simulink model "tcm"  (Simulink 8.7)
settings: Solver=ode3  StartTime=0.0  StopTime=100.0  RelTol=1e-3
undefined symbols (not defined in the file or in its folder): ap, bias, sgn
libraries: simulink x3
settings Model: Creator=mddavies  LastModifiedBy=bourbouh
settings DataIOCC: SignalLoggingSaveFormat=ModelDataLogs
settings DebuggingCC: SolverPrmCheckMsg=warning  FcnCallInpInsideContextMsg=UseLocalSettings  StateNameClashWarn=warning
settings GRTTargetCC: CombineOutputUpdateFcns=off  GRTInterface=on

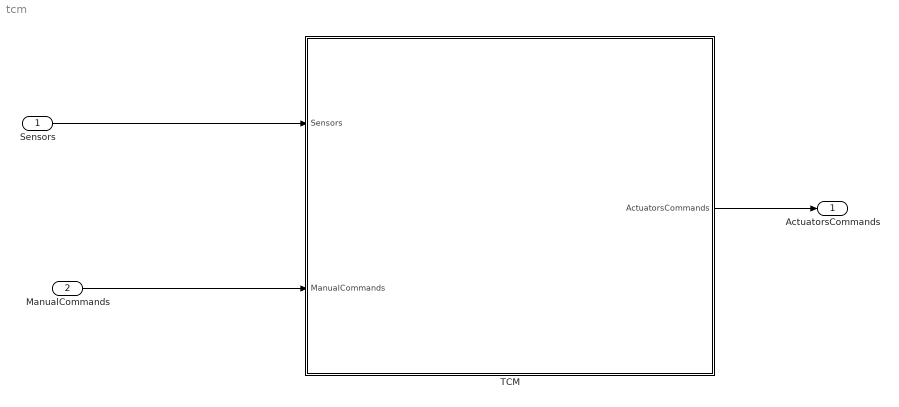
== system tcm ==
  Sensors : Inport  RequirementInfo={} %GIDa_0ce9b168_5661_42b0_b4cb_7d3faaf2df72  PortDimensions=17
  "ManualCommands " : Inport  RequirementInfo={} %GIDa_0ce9b168_5661_42b0_b4cb_7d3faaf2df72  Port=2  PortDimensions=9
  TCM : Subsystem
  ActuatorsCommands : Outport  RequirementInfo={} %GIDa_ba9bc9f0_2997_4cec_8a5a_2cb65716cddf
  wires:
  Sensors/1 -> TCM/1(Sensors)
  "ManualCommands "/1 -> TCM/2("ManualCommands ")
  TCM/1(ActuatorsCommands) -> ActuatorsCommands/1

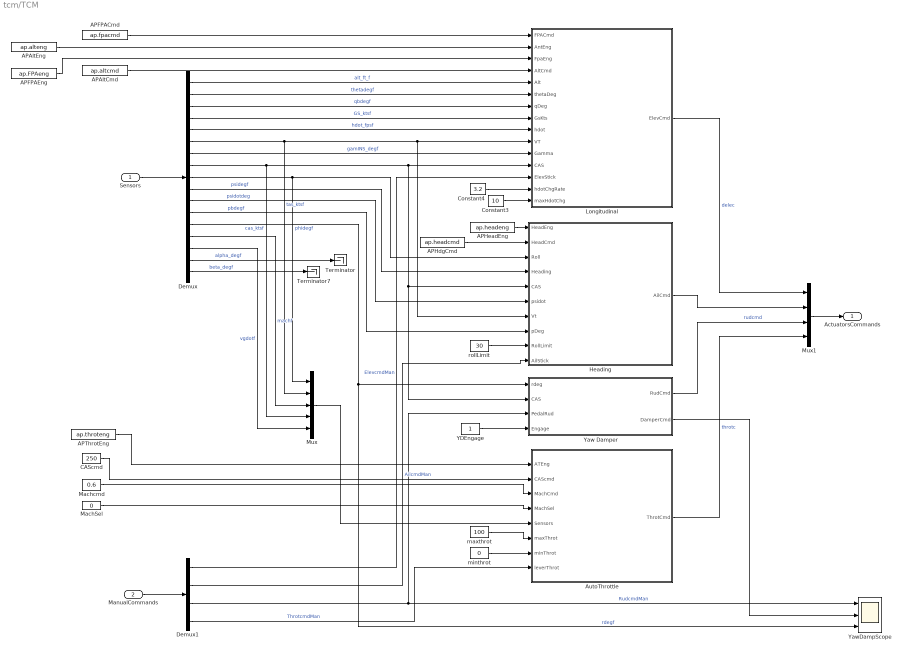
== system tcm/TCM ==
  Sensors : Inport  RequirementInfo={} %GIDa_0ce9b168_5661_42b0_b4cb_7d3faaf2df72  PortDimensions=17
  "ManualCommands " : Inport  RequirementInfo={} %GIDa_0ce9b168_5661_42b0_b4cb_7d3faaf2df72  Port=2  PortDimensions=9
  APAltCmd : Constant  RequirementInfo={} %GIDa_8396ea73_c2c1_410d_8e72_0a2c2e115229  Value=ap.altcmd
  APAltEng : Constant  RequirementInfo={} %GIDa_7acdc276_5904_4f5d_a4d8_b7eafc22dcba  Value=ap.alteng  OutDataTypeStr=boolean
  "APFPACmd " : Constant  RequirementInfo={} %GIDa_f2a9802e_c9ff_44b4_9c39_101c70e3085f  Value=ap.fpacmd
  APFPAEng : Constant  RequirementInfo={} %GIDa_b6347d6f_b14e_46b8_b79f_c4482e372009  Value=ap.FPAeng  OutDataTypeStr=boolean
  APHdgCmd : Constant  RequirementInfo={} %GIDa_ca348917_806b_4c73_b099_958ce531bbd5  Value=ap.headcmd
  APHeadEng : Constant  RequirementInfo={} %GIDa_019c8883_de5f_448b_a478_e0a40c975d97  Value=ap.headeng  OutDataTypeStr=boolean
  APThrotEng : Constant  RequirementInfo={} %GIDa_c34ca1b2_b760_48cb_8815_eaf096d766de  Value=ap.throteng  OutDataTypeStr=boolean
  AutoThrottle : Subsystem  RequirementInfo={'other' '..\..\tcm_requirements.docx' '@Simulink_requirement_item_20' 'true' 'Auto Throttle' '' } %GIDa_9e91f8aa_3697_4e86_a547_8b20eda6b794
  CAScmd : Constant  RequirementInfo={} %GIDa_47d34f1f_8d24_42cb_857b_a6284aa9b10f  Value=250
  Constant3 : Constant  RequirementInfo={} %GIDa_6046f9e1_21da_4401_862c_288f604e8689  Value=10
  Constant4 : Constant  RequirementInfo={} %GIDa_dee93be0_a932_4ef0_a207_8f7329b01ca5  Value=3.2
  Demux : Demux  Outputs=17
  Demux1 : Demux
  Heading : Subsystem
  Longitudinal : Subsystem
  MachSel : Constant  RequirementInfo={} %GIDa_703eecf9_8ffd_4677_9df1_b11ad3ff81be  Value=0
  Machcmd : Constant  RequirementInfo={} %GIDa_a015b01e_abfd_4965_a258_bc3318cb77ef  Value=0.6
  Mux : Mux  Inputs=5
  Mux1 : Mux
  Terminator : Terminator
  Terminator7 : Terminator
      settings: RequirementInfo={} %GIDa_ea750fcf_3a35_4ca3_ba61_16c7ba83d83d
  YDEngage : Constant  RequirementInfo={} %GIDa_1b340559_9c71_403c_9901_bf0a93e2b9fd  SampleTime=-1
  Yaw Damper : Subsystem  RequirementInfo={'other' '..\..\tcm_requirements.docx' '@Simulink_requirement_item_19' 'true' 'Yaw Damper' '' } %GIDa_4d9fd165_a151_41ab_8542_450c342372eb
  YawDampScope : Scope  NumInputPorts=3
      settings: RequirementInfo={} %GIDa_7592f6f2_c7e8_4acc_8768_b20cb3da46c8
  maxthrot : Constant  RequirementInfo={} %GIDa_230ab06c_3fb9_421e_bdda_8f032886ed67  Value=100  SampleTime=-1
  minthrot : Constant  RequirementInfo={} %GIDa_e24cf5cf_680d_403e_8bf4_a3705f2cf8ca  Value=0  SampleTime=-1
  rollLimit : Constant  RequirementInfo={} %GIDa_80188ac9_3eb7_4583_8db0_ebf7b7448de5  Value=30  SampleTime=-1
  ActuatorsCommands : Outport  RequirementInfo={} %GIDa_ba9bc9f0_2997_4cec_8a5a_2cb65716cddf
  wires:
  APThrotEng/1 -> AutoThrottle/1(ATEng)
  Constant4/1 -> Longitudinal/14(hdotChgRate)
  Longitudinal/1(ElevCmd) -> Mux1/1  "delec"
  Heading/1(AilCmd) -> Mux1/2
  CAScmd/1 -> AutoThrottle/2(CAScmd)
  APAltEng/1 -> Longitudinal/2(AntEng)
  Machcmd/1 -> AutoThrottle/3(MachCmd)
  MachSel/1 -> AutoThrottle/4(MachSel)
  APHeadEng/1 -> Heading/1(HeadEng)
  APFPAEng/1 -> Longitudinal/3(FpaEng)
  APHdgCmd/1 -> Heading/2(HeadCmd)
  "APFPACmd "/1 -> Longitudinal/1(FPACmd)
  APAltCmd/1 -> Longitudinal/4(AltCmd)
  maxthrot/1 -> AutoThrottle/6(maxThrot)
  Yaw Damper/2(DamperCmd) -> YawDampScope/2
  Yaw Damper/1(RudCmd) -> Mux1/3  "rudcmd"
  Constant3/1 -> Longitudinal/15(maxHdotChg)
  YDEngage/1 -> Yaw Damper/4(Engage)
  rollLimit/1 -> Heading/9(RollLimit)
  Sensors/1 -> Demux/1
  Demux/1 -> Longitudinal/5(Alt)  "alt_ft_f"
  Demux/2 -> Longitudinal/6(thetaDeg)  "thetadegf"
  Demux/4 -> Longitudinal/8(GsKts)  "GS_ktsf"
  Demux/3 -> Longitudinal/7(qDeg)  "qbdegf"
  Demux/5 -> Longitudinal/9(hdot)  "hdot_fpsf"
  Demux/6 -> Longitudinal/10(VT), Heading/7(Vt), Mux/2  "tas_ktsf"
  Demux/7 -> Longitudinal/11(Gamma)  "gamINS_degf"
  Demux/8 -> Longitudinal/12(CAS), Yaw Damper/2(CAS), Heading/5(CAS), Mux/4  "cas_ktsf"
  Demux/16 -> Terminator/1  "alpha_degf"
  Demux/17 -> Terminator7/1  "beta_degf"
  Demux/9 -> Heading/3(Roll), Mux/1  "phidegf"
  Demux/10 -> Heading/4(Heading)  "psidegf"
  Demux/11 -> Heading/6(psidot)  "psidotdeg"
  Demux/12 -> Heading/8(pDeg)  "pbdegf"
  Demux/13 -> Yaw Damper/1(rdeg), YawDampScope/3  "rdegf"
  Demux/14 -> Mux/3  "machf"
  Demux/15 -> Mux/5  "vgdotf"
  minthrot/1 -> AutoThrottle/7(minThrot)
  "ManualCommands "/1 -> Demux1/1
  Demux1/1 -> Longitudinal/13(ElevStick)  "ElevcmdMan"
  Demux1/2 -> Heading/10(AilStick)  "AilcmdMan"
  Demux1/3 -> YawDampScope/1, Yaw Damper/3(PedalRud)  "RudcmdMan"
  Demux1/4 -> AutoThrottle/8(leverThrot)  "ThrotcmdMan"
  Mux/1 -> AutoThrottle/5(Sensors)
  Mux1/1 -> ActuatorsCommands/1
  AutoThrottle/1(ThrotCmd) -> Mux1/4  "throtc"

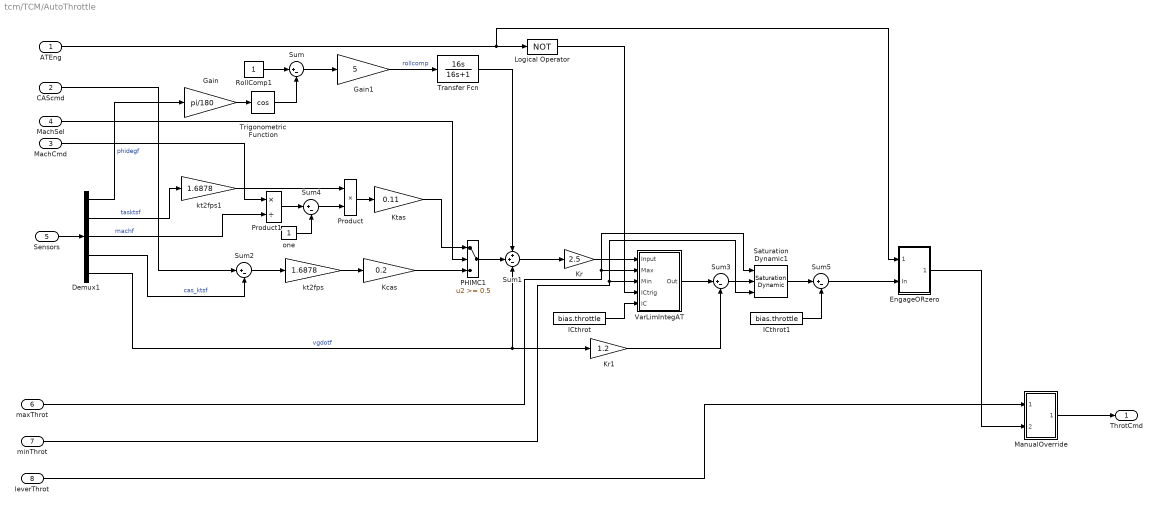
== system tcm/TCM/AutoThrottle ==
  ATEng : Inport  RequirementInfo={} %GIDa_2f45927d_6c28_4361_8173_5669474b9abd
  CAScmd : Inport  RequirementInfo={} %GIDa_92b5701d_5ed6_438c_8e94_843ad865eadf  Port=2
  MachCmd : Inport  RequirementInfo={} %GIDa_c26053c2_6b7f_4bf5_8f7d_768d0d646830  Port=3
  MachSel : Inport  RequirementInfo={} %GIDa_598b16f9_0dbe_4c96_859f_7e96536c1fb2  Port=4
  Sensors : Inport  RequirementInfo={} %GIDa_a55eff7f_fb2b_4f7a_a83b_479b402cff39  Port=5
  maxThrot : Inport  Port=6
  minThrot : Inport  Port=7
  leverThrot : Inport  Port=8
  Demux1 : Demux  Outputs=5
  EngageORzero : Subsystem
  Gain : Gain  RequirementInfo={} %GIDa_44ece66a_e9b1_47ae_9399_459633f82831  Gain=pi/180
  Gain1 : Gain  RequirementInfo={} %GIDa_5f70482a_3c80_415d_8392_528447a4813a  Gain=5
  ICthrot : Constant  RequirementInfo={} %GIDa_a96462ac_b28c_4fce_82e8_5e3952049bfb  Value=bias.throttle  SampleTime=-1
  ICthrot1 : Constant  RequirementInfo={} %GIDa_23dd534b_a590_436c_b15f_58e24838e8f2  Value=bias.throttle  SampleTime=-1
  Kcas : Gain  RequirementInfo={} %GIDa_1e6984b9_9479_49b0_970a_973f7c32edb7  Gain=0.2
  Kr : Gain  RequirementInfo={} %GIDa_18afb4c5_511e_47fb_85e5_bdfbcffb89de  Gain=2.5
  Kr1 : Gain  RequirementInfo={} %GIDa_9e9297b4_8c75_4533_a8dd_3891075538e5  Gain=1.2
  Ktas : Gain  RequirementInfo={} %GIDa_43c0fedf_b3e4_4e0f_a6fc_568c741b4ee2  Gain=0.11
  Logical Operator : Logic  RequirementInfo={} %GIDa_18e0a705_4fb5_4f14_a12b_8f6e047bc903  Operator=NOT  AllPortsSameDT=off  OutDataTypeStr=boolean
  ManualOverride : Subsystem
  PHIMC1 : Switch  RequirementInfo={} %GIDa_e2112eb0_c2db_4683_9846_bc0eb97a67f4  Threshold=0.5  SampleTime=0.02  SaturateOnIntegerOverflow=on
  Product : Product  RequirementInfo={} %GIDa_f2e51a99_89d7_4199_acd2_75b4a5a762fd  RndMeth=Zero
  Product1 : Product  RequirementInfo={} %GIDa_5c94e278_e588_4429_922d_3903b6601868  Inputs=*/  RndMeth=Zero
  RollComp1 : Constant  RequirementInfo={} %GIDa_8f810878_51f3_4d16_a407_aaec8ff4cd8a  SampleTime=-1
  Saturation Dynamic1 : simulink/Discontinuities/Saturation Dynamic  OutMin=[]  OutMax=[]  OutDataTypeStr=Inherit: Same as second input  OutDataType=sfix(16)  OutScaling=2^-10  DoSatur=off
  Sum : Sum  RequirementInfo={} %GIDa_9c88a12f_8eea_40db_a15a_aac24376aa7e  Inputs=|+-
  Sum1 : Sum  RequirementInfo={} %GIDa_fc0b036c_eb6d_4b0a_a40d_b7183183f1bc  Inputs=++-
  Sum2 : Sum  RequirementInfo={} %GIDa_95fcf8e7_99a7_46b3_9e41_77bfb2af0e6e  Inputs=|+-
  Sum3 : Sum  RequirementInfo={} %GIDa_0620e5c6_0d29_4c42_bdd5_2c680788712f  Inputs=|+-
  Sum4 : Sum  RequirementInfo={} %GIDa_a4cfd5ae_8cc7_4a4b_9229_0e28a225e0c7  Inputs=|+-
  Sum5 : Sum  RequirementInfo={} %GIDa_9cd0e9e4_7a0b_4a48_8c2a_57da4ad43678  Inputs=|+-
  Transfer Fcn : TransferFcn  RequirementInfo={} %GIDa_76b9b3a6_995f_4f78_b7a2_a7361be06aec  Numerator=[16 0]  Denominator=[16 1]
  Trigonometric Function : Trigonometry  RequirementInfo={} %GIDa_82d3b8e2_fba4_4fde_a324_6f5a5fa38b0e  Operator=cos
  VarLimIntegAT : Subsystem  RequirementInfo={} %GIDa_946bbead_442f_495f_943e_e8a8eb5a05a2
  kt2fps : Gain  RequirementInfo={} %GIDa_719dda5c_99e9_4155_8171_b1c9b5878f3a  Gain=1.6878
  kt2fps1 : Gain  RequirementInfo={} %GIDa_b06df2d8_ff63_4d20_83d9_1b3d18a391c7  Gain=1.6878
  one : Constant  RequirementInfo={} %GIDa_79530773_343c_40ed_88d6_a702a3c8b7d7  SampleTime=-1
  ThrotCmd : Outport  RequirementInfo={} %GIDa_10832092_f513_4063_bf4d_710db5c9192f
  wires:
  CAScmd/1 -> Sum2/1
  Sum2/1 -> kt2fps/1
  Sum1/1 -> Kr/1
  kt2fps/1 -> Kcas/1
  Kr/1 -> VarLimIntegAT/1(Input)
  Kr1/1 -> Sum3/2
  Gain1/1 -> Transfer Fcn/1  "rollcomp"
  Sum/1 -> Gain1/1
  Trigonometric Function/1 -> Sum/2
  RollComp1/1 -> Sum/1
  Gain/1 -> Trigonometric Function/1
  Product1/1 -> Sum4/1
  one/1 -> Sum4/2
  Sum4/1 -> Product/2
  kt2fps1/1 -> Product/1
  Product/1 -> Ktas/1
  ICthrot/1 -> VarLimIntegAT/5(IC)
  Sum5/1 -> EngageORzero/2(In)
  ICthrot1/1 -> Sum5/2
  maxThrot/1 -> VarLimIntegAT/2(Max), Saturation Dynamic1/1
  minThrot/1 -> VarLimIntegAT/3(Min), Saturation Dynamic1/3
  VarLimIntegAT/1(Out) -> Sum3/1
  Sum3/1 -> Saturation Dynamic1/2
  Saturation Dynamic1/1 -> Sum5/1
  PHIMC1/1 -> Sum1/2
  Kcas/1 -> PHIMC1/3
  Ktas/1 -> PHIMC1/1
  Transfer Fcn/1 -> Sum1/1
  Logical Operator/1 -> VarLimIntegAT/4(ICtrig)
  ATEng/1 -> EngageORzero/1(Engage), Logical Operator/1
  MachSel/1 -> PHIMC1/2
  MachCmd/1 -> Product1/1
  leverThrot/1 -> ManualOverride/1(Man)
  ManualOverride/1(Out) -> ThrotCmd/1
  EngageORzero/1(Out) -> ManualOverride/2(Auto)
  Sensors/1 -> Demux1/1
  Demux1/1 -> Gain/1  "phidegf"
  Demux1/2 -> kt2fps1/1  "tasktsf"
  Demux1/3 -> Product1/2  "machf"
  Demux1/4 -> Sum2/2  "cas_ktsf"
  Demux1/5 -> Sum1/3, Kr1/1  "vgdotf"

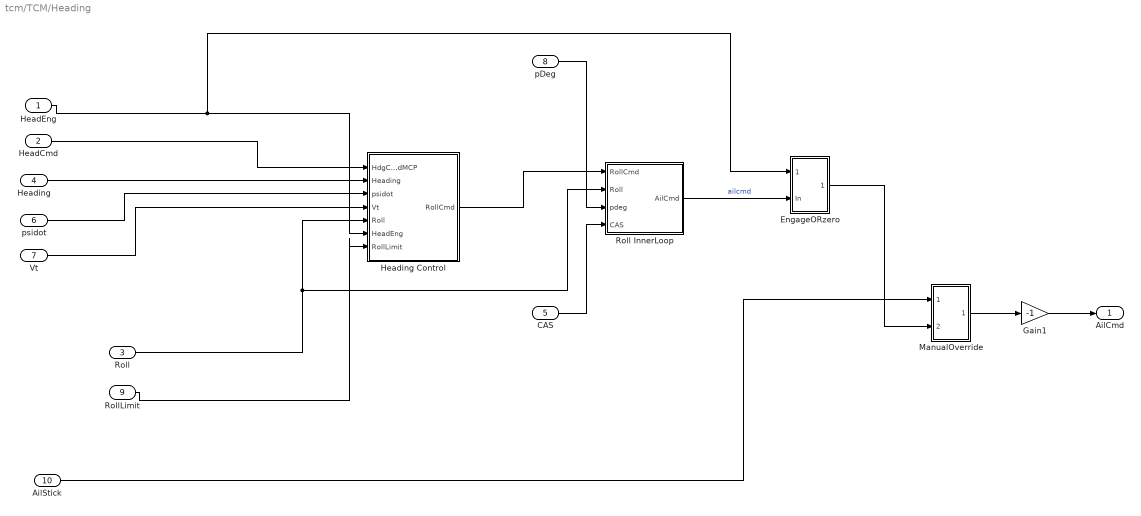
== system tcm/TCM/Heading ==
  HeadEng : Inport
  HeadCmd : Inport  Port=2
  Roll : Inport  Port=3
  Heading : Inport  Port=4
  CAS : Inport  Port=5
  psidot : Inport  Port=6
  Vt : Inport  Port=7
  pDeg : Inport  Port=8
  RollLimit : Inport  Port=9
  AilStick : Inport  Port=10
  EngageORzero : Subsystem
  Gain1 : Gain  RequirementInfo={} %GIDa_2f421c02_996e_46c9_ac2a_3c25b016b229  Gain=-1  SaturateOnIntegerOverflow=on  OutDataTypeStr=Inherit: Same as input  ParamDataTypeStr=Inherit: Same as input
  Heading Control : Subsystem  RequirementInfo={'other' '..\..\tcm_requirements.docx' '@Simulink_requirement_item_16' 'true' 'Heading Control' '' } %GIDa_911b8f78_7600_4481_9e93_a11b2a64dbe5
  ManualOverride : Subsystem
  Roll InnerLoop : Subsystem  RequirementInfo={'other' '..\..\tcm_requirements.docx' '@Simulink_requirement_item_18' 'true' 'Roll InnerLoop' '' } %GIDa_311280c1_10c2_4ab3_a776_5e785b9037f8
  AilCmd : Outport
  wires:
  pDeg/1 -> Roll InnerLoop/3(pdeg)
  Vt/1 -> Heading Control/4(Vt)
  psidot/1 -> Heading Control/3(psidot)
  Heading/1 -> Heading Control/2(Heading)
  Roll/1 -> Heading Control/5(Roll), Roll InnerLoop/2(Roll)
  Heading Control/1(RollCmd) -> Roll InnerLoop/1(RollCmd)
  Roll InnerLoop/1(AilCmd) -> EngageORzero/2(In)  "ailcmd"
  HeadCmd/1 -> Heading Control/1(HdgCmdMCP)
  HeadEng/1 -> EngageORzero/1(Engage), Heading Control/6(HeadEng)
  CAS/1 -> Roll InnerLoop/4(CAS)
  RollLimit/1 -> Heading Control/7(RollLimit)
  ManualOverride/1(Out) -> Gain1/1
  AilStick/1 -> ManualOverride/1(Man)
  Gain1/1 -> AilCmd/1
  EngageORzero/1(Out) -> ManualOverride/2(Auto)

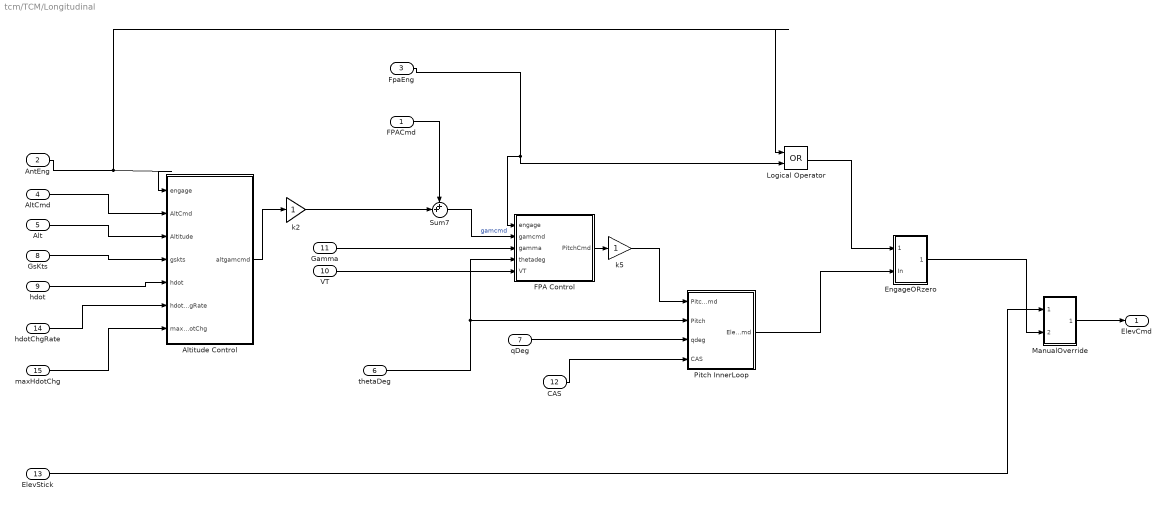
== system tcm/TCM/Longitudinal ==
  FPACmd : Inport
  AntEng : Inport  Port=2
  FpaEng : Inport  Port=3
  AltCmd : Inport  Port=4
  Alt : Inport  Port=5
  thetaDeg : Inport  Port=6
  qDeg : Inport  Port=7
  GsKts : Inport  Port=8
  hdot : Inport  Port=9
  VT : Inport  Port=10
  Gamma : Inport  Port=11
  CAS : Inport  Port=12
  ElevStick : Inport  Port=13
  hdotChgRate : Inport  Port=14
  maxHdotChg : Inport  Port=15
  Altitude Control : Subsystem  RequirementInfo={'other' '..\..\tcm_requirements.docx' '@Simulink_requirement_item_14' 'true' 'Altitude Control' '' } %GIDa_440f81f7_8b55_4c78_bea7_52c909831264
  EngageORzero : Subsystem
  FPA Control : Subsystem  RequirementInfo={'other' '..\..\tcm_requirements.docx' '@Simulink_requirement_item_15' 'true' 'FPA Control' '' } %GIDa_71e3e321_cc66_4d8a_a4f3_fd2e7f1fbaff
  Logical Operator : Logic  Operator=OR  AllPortsSameDT=off  OutDataTypeStr=boolean
  ManualOverride : Subsystem
  Pitch InnerLoop : Subsystem  RequirementInfo={'other' '..\..\tcm_requirements.docx' '@Simulink_requirement_item_17' 'true' 'Pitch InnerLoop' '' } %GIDa_fc56dd5e_d6cd_42fe_934f_e4aed2c76eb1
  Sum7 : Sum  RequirementInfo={} %GIDa_92495686_3877_4412_b19f_22e099e095ee  Inputs=++|
  k2 : Gain  RequirementInfo={} %GIDa_7e514706_5da4_4f1f_bf6c_0050dd9ce76d
  k5 : Gain  RequirementInfo={} %GIDa_b8b0ba7d_7fd3_4b03_b740_56530c3187c8
  ElevCmd : Outport
  wires:
  k2/1 -> Sum7/2
  Alt/1 -> Altitude Control/3(Altitude)
  thetaDeg/1 -> FPA Control/4(thetadeg), Pitch InnerLoop/2(Pitch)
  Gamma/1 -> FPA Control/3(gamma)
  AltCmd/1 -> Altitude Control/2(AltCmd)
  ManualOverride/1(Out) -> ElevCmd/1
  Altitude Control/1(altgamcmd) -> k2/1
  FPA Control/1(PitchCmd) -> k5/1
  hdot/1 -> Altitude Control/5(hdot)
  Sum7/1 -> FPA Control/2(gamcmd)  "gamcmd"
  qDeg/1 -> Pitch InnerLoop/3(qdeg)
  GsKts/1 -> Altitude Control/4(gskts)
  VT/1 -> FPA Control/5(VT)
  FPACmd/1 -> Sum7/1
  k5/1 -> Pitch InnerLoop/1(PitchCmd)
  FpaEng/1 -> Logical Operator/2, FPA Control/1(engage)
  CAS/1 -> Pitch InnerLoop/4(CAS)
  AntEng/1 -> Logical Operator/1, Altitude Control/1(engage)
  ElevStick/1 -> ManualOverride/1(Man)
  Pitch InnerLoop/1(ElevCmd) -> EngageORzero/2(In)
  EngageORzero/1(Out) -> ManualOverride/2(Auto)
  Logical Operator/1 -> EngageORzero/1(Engage)
  maxHdotChg/1 -> Altitude Control/7(maxHdotChg)
  hdotChgRate/1 -> Altitude Control/6(hdotChgRate)

== system tcm/TCM/Yaw Damper ==
  rdeg : Inport  RequirementInfo={} %GIDa_aab456ca_baa8_40be_af7c_3007e2406789
  CAS : Inport  RequirementInfo={} %GIDa_ffc3df4d_90ed_429c_9905_ba1d5e1c6104  Port=2
  PedalRud : Inport  Port=3
  Engage : Inport  Port=4
  EngageORzero : Subsystem
  Kcas : Lookup  RequirementInfo={} %GIDa_a54aaa82_92c8_4b54_937a_3aadc5cc777a  InputValues=[0 120 350 500]  Table=[1.0 1.0 0.3 0.3]
  Kr : Gain  RequirementInfo={} %GIDa_e1600aee_198d_416e_b040_c3f06ae50aaa  Gain=1.25
  ManualOverride : Subsystem
  Product : Product  RequirementInfo={} %GIDa_b93a6279_44c9_4030_b746_3332e584ca8b  RndMeth=Zero
  YD_wo : TransferFcn  RequirementInfo={} %GIDa_e4ecddaf_b3d8_4a89_aabe_57315209a16f  Numerator=[1 0]  Denominator=[1 10]
  RudCmd : Outport  RequirementInfo={} %GIDa_5d934514_ad75_43c8_8562_5e4d07d2a065
  DamperCmd : Outport  Port=2
  wires:
  rdeg/1 -> Kr/1
  CAS/1 -> Kcas/1
  Kcas/1 -> Product/2
  ManualOverride/1(Out) -> RudCmd/1
  Kr/1 -> YD_wo/1
  YD_wo/1 -> Product/1
  EngageORzero/1(Out) -> ManualOverride/2(Auto), DamperCmd/1
  PedalRud/1 -> ManualOverride/1(Man)
  Engage/1 -> EngageORzero/1(Engage)
  Product/1 -> EngageORzero/2(In)

== system tcm/TCM/AutoThrottle/EngageORzero ==
  Engage : Inport
  In : Inport  Port=2
  Logical Operator5 : Logic  RequirementInfo={} %GIDa_13e72d9c_1630_4494_8181_04ea596767a9  AllPortsSameDT=off  OutDataTypeStr=boolean
  Switch1 : Switch  RequirementInfo={} %GIDa_d89bdcfc_1e33_494f_b3fe_e13e317b4b5d  Threshold=0.5
  zero10 : Constant  RequirementInfo={} %GIDa_d1e784f7_2146_48f6_874a_0add9f175ac2
  zero9 : Constant  RequirementInfo={} %GIDa_df8b3a8b_00d1_4891_87af_e83379ed0682  Value=0
  Out : Outport
  wires:
  Engage/1 -> Logical Operator5/1
  zero10/1 -> Logical Operator5/2
  zero9/1 -> Switch1/3
  In/1 -> Switch1/1
  Logical Operator5/1 -> Switch1/2
  Switch1/1 -> Out/1

== system tcm/TCM/AutoThrottle/ManualOverride ==
  Man : Inport
  Auto : Inport  Port=2
  Switch1 : Switch  RequirementInfo={} %GIDa_99412258_89e8_4c84_a7a6_8adb3817b9de  Criteria=u2 ~= 0  Threshold=0.5
  Out : Outport
  wires:
  Man/1 -> Switch1/3, Switch1/2
  Auto/1 -> Switch1/1
  Switch1/1 -> Out/1

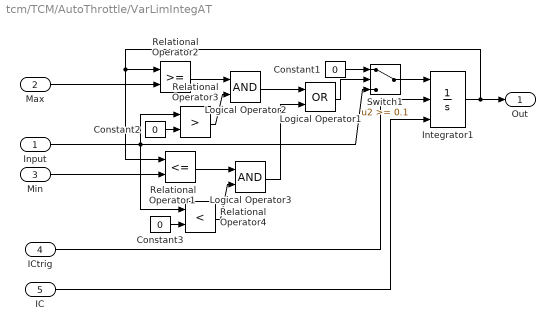
== system tcm/TCM/AutoThrottle/VarLimIntegAT ==
  Input : Inport  RequirementInfo={} %GIDa_91b38f96_ed38_45a6_8bb9_ff3fb81525df
  Max : Inport  RequirementInfo={} %GIDa_5200ce52_bb44_458c_9945_e382c2e773b4  Port=2
  Min : Inport  RequirementInfo={} %GIDa_600874e9_d5fd_4de5_b948_9284e9d56639  Port=3
  ICtrig : Inport  RequirementInfo={} %GIDa_af678c0a_424b_44b8_aa3a_3f303d846e8e  Port=4
  IC : Inport  RequirementInfo={} %GIDa_872b1a96_8436_4d34_8580_74ad3366301d  Port=5
  Constant1 : Constant  RequirementInfo={} %GIDa_bf704cc0_6bc9_4624_9fa4_e77befe43ee9  Value=0  SampleTime=-1
  Constant2 : Constant  RequirementInfo={} %GIDa_7032ed75_2ad3_41e5_9584_0891c369141c  Value=0  SampleTime=-1
  Constant3 : Constant  RequirementInfo={} %GIDa_f4367f96_4d82_41b7_8e43_0c6cec23a023  Value=0  SampleTime=-1
  Integrator1 : Integrator  RequirementInfo={} %GIDa_d4336f3d_c52f_4cf1_85ef_86b185e703b9  ExternalReset=level  InitialConditionSource=external
  Logical Operator1 : Logic  RequirementInfo={} %GIDa_53e2ecf2_1671_4b86_a4e6_7e9f03594f4a  Operator=OR
  Logical Operator2 : Logic  RequirementInfo={} %GIDa_f9639a17_73a7_4a19_b9c3_2b3e1bcf1152
  Logical Operator3 : Logic  RequirementInfo={} %GIDa_53705a9e_f0e6_4df8_b74a_51dda5b71ea0
  Relational Operator1 : RelationalOperator  RequirementInfo={} %GIDa_85cee0a0_d47b_41e2_b8dd_f48b296f5cf4  Operator=<=  InputSameDT=on
  Relational Operator2 : RelationalOperator  RequirementInfo={} %GIDa_74942223_cbc1_42b5_8e5e_e6b9112f9130  InputSameDT=on
  Relational Operator3 : RelationalOperator  RequirementInfo={} %GIDa_ea1202bb_7a42_4314_84fa_c36aa79c966a  Operator=>  InputSameDT=on
  Relational Operator4 : RelationalOperator  RequirementInfo={} %GIDa_c9e3adfb_bd3d_4cfe_9bd6_4a3fd1707fe2  Operator=<  InputSameDT=on
  Switch1 : Switch  RequirementInfo={} %GIDa_ed603307_5c4b_4569_8f05_95ce39b1df88  Threshold=0.1  SaturateOnIntegerOverflow=on  InputSameDT=on
  Out : Outport  RequirementInfo={} %GIDa_a7cb998d_eb28_45ce_8ac9_f1554f32fe4e
  wires:
  IC/1 -> Integrator1/3
  ICtrig/1 -> Integrator1/2
  Min/1 -> Relational Operator1/2
  Max/1 -> Relational Operator2/2
  Constant3/1 -> Relational Operator4/2
  Input/1 -> Switch1/3, Relational Operator3/1, Relational Operator4/1
  Logical Operator3/1 -> Logical Operator1/2
  Relational Operator4/1 -> Logical Operator3/2
  Relational Operator1/1 -> Logical Operator3/1
  Constant2/1 -> Relational Operator3/2
  Logical Operator2/1 -> Logical Operator1/1
  Relational Operator3/1 -> Logical Operator2/2
  Relational Operator2/1 -> Logical Operator2/1
  Logical Operator1/1 -> Switch1/2
  Integrator1/1 -> Relational Operator2/1, Relational Operator1/1, Out/1
  Switch1/1 -> Integrator1/1
  Constant1/1 -> Switch1/1

== system tcm/TCM/Heading/EngageORzero ==
  Engage : Inport
  In : Inport  Port=2
  Logical Operator5 : Logic  RequirementInfo={} %GIDa_7add67f6_200e_4459_8afc_a50a3802c341  AllPortsSameDT=off  OutDataTypeStr=boolean
  Switch1 : Switch  RequirementInfo={} %GIDa_a1777089_6daf_41d2_9e69_9356c4782e25  Threshold=0.5
  zero10 : Constant  RequirementInfo={} %GIDa_d889400f_b153_4cfc_a180_15b84145f1e0
  zero9 : Constant  RequirementInfo={} %GIDa_9027fd24_3b48_4acd_a774_517fb1aa3516  Value=0
  Out : Outport
  wires:
  Engage/1 -> Logical Operator5/1
  zero10/1 -> Logical Operator5/2
  zero9/1 -> Switch1/3
  In/1 -> Switch1/1
  Logical Operator5/1 -> Switch1/2
  Switch1/1 -> Out/1

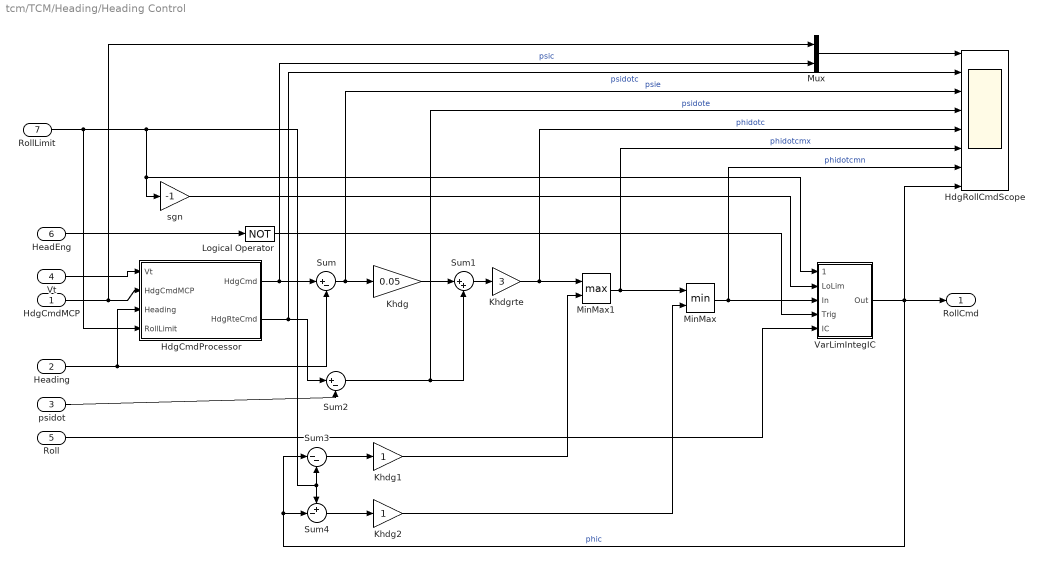
== system tcm/TCM/Heading/Heading Control ==
  HdgCmdMCP : Inport  RequirementInfo={} %GIDa_afcd05d1_a9dc_45a7_a8f8_7136ccc61726
  Heading : Inport  RequirementInfo={} %GIDa_19b80fe4_d265_482c_b709_18db80a7cdf3  Port=2
  psidot : Inport  RequirementInfo={} %GIDa_e421e82d_0cc7_4ad7_ac7a_9fb430d189d5  Port=3
  Vt : Inport  RequirementInfo={} %GIDa_9daf3e20_e00e_4f36_b534_d9747a241338  Port=4
  Roll : Inport  RequirementInfo={} %GIDa_8629ba77_a751_4097_af53_617eaa1017be  Port=5
  HeadEng : Inport  RequirementInfo={} %GIDa_dadb1310_2bf4_48cf_8970_85174d784ee3  Port=6
  RollLimit : Inport  Port=7
  HdgCmdProcessor : Subsystem  RequirementInfo={} %GIDa_3cb77e5f_f630_4f22_88a8_7528bfceb83f
  HdgRollCmdScope : Scope  NumInputPorts=8
      settings: RequirementInfo={} %GIDa_5fbe2135_fdf1_4f64_a179_faa1710ae21e
  Khdg : Gain  RequirementInfo={} %GIDa_abf81b08_c210_4343_b4da_5a7e229caeb6  Gain=0.05
  Khdg1 : Gain  RequirementInfo={} %GIDa_7a7a35ca_24a5_4d20_bc30_55deea16462c
  Khdg2 : Gain  RequirementInfo={} %GIDa_57191899_7ee5_4454_897a_7009651ed5fb
  Khdgrte : Gain  RequirementInfo={} %GIDa_bcc6a420_18f3_43f0_aaa1_aaa1bbf90f64  Gain=3
  Logical Operator : Logic  RequirementInfo={} %GIDa_5ad405ac_0a88_4b96_aa0e_75483351ee25  Operator=NOT  AllPortsSameDT=off  OutDataTypeStr=boolean
  MinMax : MinMax  RequirementInfo={} %GIDa_4b9381d8_eb85_418b_a975_85846d5ca8c2  Inputs=2
  MinMax1 : MinMax  RequirementInfo={} %GIDa_b40e082d_0fb2_4088_baf4_e9a71be9bcc1  Function=max  Inputs=2
  Mux : Mux  RequirementInfo={} %GIDa_0e83f6c6_ae04_43dd_95fe_a79ec32b40e2  Inputs=2
  Sum : Sum  RequirementInfo={} %GIDa_b89885fc_f86c_4a50_8ce5_47d0488bdc1c  Inputs=|+-
  Sum1 : Sum  RequirementInfo={} %GIDa_40ec6862_b1f8_4f97_ae14_1eadabbceb30  Inputs=|++
  Sum2 : Sum  RequirementInfo={} %GIDa_307d6880_3ab8_4deb_90e0_d68f11d87c85  Inputs=|+-
  Sum3 : Sum  RequirementInfo={} %GIDa_ebb8b765_7f4a_435f_be61_680d3199141b  Inputs=|--
  Sum4 : Sum  RequirementInfo={} %GIDa_05638559_562a_476e_9e4c_91124434a43b  Inputs=+-|
  VarLimIntegIC : Subsystem  RequirementInfo={} %GIDa_7da7eaf5_9731_498e_9aad_b41279918004
  sgn : Gain  RequirementInfo={} %GIDa_84e2dc00_f2e5_41f4_89ce_c9fef234974f  Gain=-1
  RollCmd : Outport  RequirementInfo={} %GIDa_aa862f7f_5d4e_408f_b8c4_26b4ce96fbda
  wires:
  Heading/1 -> Sum/2, HdgCmdProcessor/3(Heading)
  HdgCmdProcessor/1(HdgCmd) -> Sum/1, Mux/2  "psic"
  Sum/1 -> Khdg/1, HdgRollCmdScope/3  "psie"
  Khdg/1 -> Sum1/1
  Sum2/1 -> Sum1/2, HdgRollCmdScope/4  "psidote"
  HdgCmdProcessor/2(HdgRteCmd) -> Sum2/1, HdgRollCmdScope/2  "psidotc"
  psidot/1 -> Sum2/2
  Vt/1 -> HdgCmdProcessor/1(Vt)
  HdgCmdMCP/1 -> HdgCmdProcessor/2(HdgCmdMCP), Mux/1
  VarLimIntegIC/1(Out) -> RollCmd/1, Sum3/1, Sum4/2, HdgRollCmdScope/8  "phic"
  RollLimit/1 -> HdgCmdProcessor/4(RollLimit), Sum4/1, Sum3/2, VarLimIntegIC/1(UpLim), sgn/1
  sgn/1 -> VarLimIntegIC/2(LoLim)
  Sum1/1 -> Khdgrte/1
  MinMax1/1 -> MinMax/1, HdgRollCmdScope/6  "phidotcmx"
  MinMax/1 -> VarLimIntegIC/3(In), HdgRollCmdScope/7  "phidotcmn"
  HeadEng/1 -> Logical Operator/1
  Sum3/1 -> Khdg1/1
  Sum4/1 -> Khdg2/1
  Khdg1/1 -> MinMax1/2
  Khdg2/1 -> MinMax/2
  Roll/1 -> VarLimIntegIC/5(IC)
  Khdgrte/1 -> MinMax1/1, HdgRollCmdScope/5  "phidotc"
  Logical Operator/1 -> VarLimIntegIC/4(Trig)
  Mux/1 -> HdgRollCmdScope/1

== system tcm/TCM/Heading/ManualOverride ==
  Man : Inport
  Auto : Inport  Port=2
  Switch1 : Switch  RequirementInfo={} %GIDa_5800ea93_45af_42da_974c_4cd975d0b8c8  Criteria=u2 ~= 0  Threshold=0.5
  Out : Outport
  wires:
  Man/1 -> Switch1/3, Switch1/2
  Auto/1 -> Switch1/1
  Switch1/1 -> Out/1

== system tcm/TCM/Heading/Roll InnerLoop ==
  note: orig =[0 60 140]
  note: orig = 0.25
  note: orig = 0.8
  RollCmd : Inport  RequirementInfo={} %GIDa_549f9d91_ca5c_4ec7_bf56_cf05f3793396
  Roll : Inport  RequirementInfo={} %GIDa_d885705c_af8c_4e18_b4d1_2f073687ea2c  Port=2
  pdeg : Inport  RequirementInfo={} %GIDa_ba7aa095_15b8_4f85_9051_8b947d28a24d  Port=3
  CAS : Inport  RequirementInfo={} %GIDa_defe4f55_1722_479a_b684_dc07a497c4ef  Port=4
  Kcas : Lookup  RequirementInfo={} %GIDa_a4bb01cf_3e83_4399_bf23_48aae96637bb  InputValues=[0 120 350 500]  Table=[1.0 1.0 0.3 0.3]
  Kphierr : Gain  RequirementInfo={} %GIDa_96c602a9_a07d_4519_9a2c_04c20a8c958d  Gain=0.5
  Product : Product  RequirementInfo={} %GIDa_6029a1e1_bbec_4e58_a2a6_3f9df62d6e90  RndMeth=Zero
  Roll_IL_scope : Scope  NumInputPorts=7
      settings: RequirementInfo={} %GIDa_ec5ee575_c049_4397_a5dd_5347629f97a6
  Sum : Sum  RequirementInfo={} %GIDa_6dd565f9_cc9c_463a_985b_c182e040d7fd  Inputs=|+-
  Sum1 : Sum  RequirementInfo={} %GIDa_02561aa6_0360_4e6c_b76e_5dde7f2ab3b1  Inputs=|+-
  rollrate_IL : ZeroPole  RequirementInfo={} %GIDa_636569be_bc7e_4244_84a4_4a62b7fc0808  Zeros=0  Poles=-0.5  Gain=0.00645
  AilCmd : Outport  RequirementInfo={} %GIDa_cd7ddcd8_c7c7_43e2_be4e_2c0bb3f4c702
  wires:
  Product/1 -> AilCmd/1, Roll_IL_scope/6  "ailcmd"
  Kcas/1 -> Product/2, Roll_IL_scope/7  "kcas"
  Sum1/1 -> Product/1
  CAS/1 -> Kcas/1
  rollrate_IL/1 -> Sum1/2, Roll_IL_scope/5  "pdegwo"
  pdeg/1 -> rollrate_IL/1, Roll_IL_scope/4  "pdeg"
  Kphierr/1 -> Sum1/1
  Roll/1 -> Sum/2, Roll_IL_scope/2  "roll"
  Sum/1 -> Kphierr/1, Roll_IL_scope/3  "rollerr"
  RollCmd/1 -> Sum/1, Roll_IL_scope/1  "rollcmd"

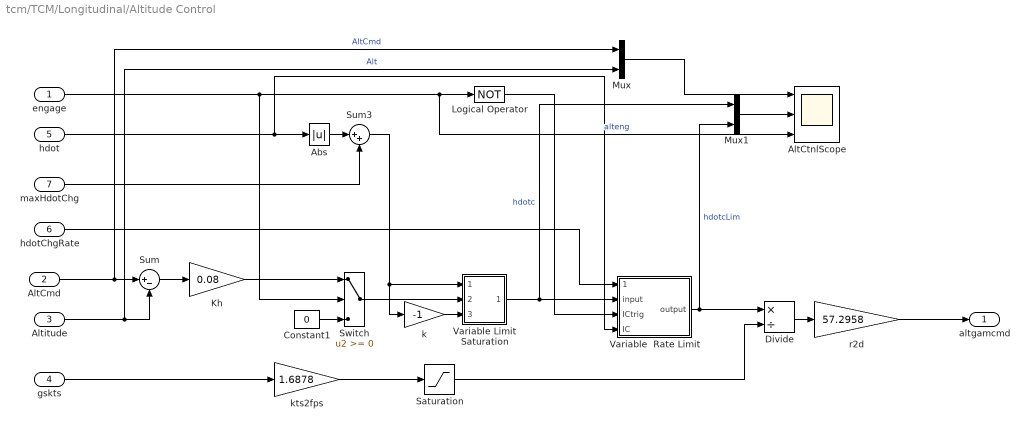
== system tcm/TCM/Longitudinal/Altitude Control ==
  engage : Inport  RequirementInfo={} %GIDa_92edc9e2_4cfd_4b16_8fee_8b94964575da
  AltCmd : Inport  RequirementInfo={} %GIDa_edbc7e5c_23e1_4d8f_98c5_e2d77895a510  Port=2
  Altitude : Inport  RequirementInfo={} %GIDa_01b40abf_ece8_4194_aeed_7639b2f9d320  Port=3
  gskts : Inport  RequirementInfo={} %GIDa_49aaf918_ec6b_4cc9_bdad_efb02f39ea3b  Port=4
  hdot : Inport  RequirementInfo={} %GIDa_f8353919_6ca2_40ed_9884_9c34b61b1365  Port=5
  hdotChgRate : Inport  Port=6
  maxHdotChg : Inport  Port=7
  Abs : Abs  RequirementInfo={} %GIDa_1391aa7c_5846_4be5_914e_111d8f2c4215  SaturateOnIntegerOverflow=on
  AltCtnlScope : Scope  NumInputPorts=3
      settings: RequirementInfo={} %GIDa_baad481c_a27b_41ac_bf32_d6e1a7f2cfe1
  Constant1 : Constant  RequirementInfo={} %GIDa_566c4b52_316f_4d36_82bb_fb65e53f78d2  Value=0
  Divide : Product  RequirementInfo={} %GIDa_b9d1a3fe_7e00_46b2_9426_cf952dcaf391  Inputs=*/
  Kh : Gain  RequirementInfo={} %GIDa_de6b2d53_b3f4_42e2_83e9_439be9ccc299  Gain=0.08
  Logical Operator : Logic  RequirementInfo={} %GIDa_921e6188_0ac2_4a9c_befc_5c7a6835e9e6  Operator=NOT
  Mux : Mux  RequirementInfo={} %GIDa_68aa779e_2c07_4c3b_9ca1_0ecb3161e49a  Inputs=2
  Mux1 : Mux  RequirementInfo={} %GIDa_0a0909f8_d09a_4568_9828_3f29982a74b3  Inputs=2
  Saturation : Saturate  RequirementInfo={} %GIDa_77166b67_e163_40e1_b7e4_7e7410a56d29  UpperLimit=1000  LowerLimit=0.0001
  Sum : Sum  RequirementInfo={} %GIDa_d94a0856_9d8d_4fca_8b77_5f1cf21c0c3a  Inputs=|+-
  Sum3 : Sum  RequirementInfo={} %GIDa_3ee7802b_411f_4586_886f_8bdef6cfccb9  Inputs=|++  SaturateOnIntegerOverflow=on  InputSameDT=on  OutDataTypeStr=Inherit: Same as first input
  Switch : Switch  RequirementInfo={} %GIDa_64af29d5_be60_4de8_bcf5_833ab8e70f35
  Variable  Rate Limit : Subsystem  RequirementInfo={} %GIDa_7d0e1926_4469_4591_916e_2bb88ddee008
  Variable Limit Saturation : Subsystem  RequirementInfo={} %GIDa_0b931211_59c1_4508_94b8_12d4cca2cb6b
  k : Gain  RequirementInfo={} %GIDa_65a0c0b6_6e9b_4a97_b326_1d79079cc625  Gain=-1
  kts2fps : Gain  RequirementInfo={} %GIDa_a49848e7_9841_44de_8ec7_08f1ed28d1e0  Gain=1.6878
  r2d : Gain  RequirementInfo={} %GIDa_934ba914_aaac_471d_9b5e_a120031a3853  Gain=57.2958
  altgamcmd : Outport  RequirementInfo={} %GIDa_3c331913_004d_4e8f_a0a1_b052c80c7670
  wires:
  Sum/1 -> Kh/1
  AltCmd/1 -> Sum/1, Mux/1  "AltCmd"
  Altitude/1 -> Sum/2, Mux/2  "Alt"
  hdot/1 -> Abs/1, Variable  Rate Limit/4(IC)
  Abs/1 -> Sum3/1
  maxHdotChg/1 -> Sum3/2
  k/1 -> Variable Limit Saturation/3(Lo_lim)
  Sum3/1 -> k/1, Variable Limit Saturation/1(up_lim)
  engage/1 -> Switch/2, Logical Operator/1, AltCtnlScope/3  "alteng"
  gskts/1 -> kts2fps/1
  Divide/1 -> r2d/1
  r2d/1 -> altgamcmd/1
  Logical Operator/1 -> Variable  Rate Limit/3(ICtrig)
  Variable Limit Saturation/1(Out1) -> Variable  Rate Limit/2(input), Mux1/1  "hdotc"
  hdotChgRate/1 -> Variable  Rate Limit/1(ratelim)
  Variable  Rate Limit/1(output) -> Divide/1, Mux1/2  "hdotcLim"
  kts2fps/1 -> Saturation/1
  Saturation/1 -> Divide/2
  Switch/1 -> Variable Limit Saturation/2(SigIn)
  Kh/1 -> Switch/1
  Constant1/1 -> Switch/3
  Mux/1 -> AltCtnlScope/1
  Mux1/1 -> AltCtnlScope/2

== system tcm/TCM/Longitudinal/EngageORzero ==
  Engage : Inport
  In : Inport  Port=2
  Logical Operator5 : Logic  RequirementInfo={} %GIDa_2faaa958_fdd5_4161_8224_87bc655595ec  AllPortsSameDT=off  OutDataTypeStr=boolean
  Switch1 : Switch  RequirementInfo={} %GIDa_cd8505b1_f38c_41a3_a83c_5e083797b181  Threshold=0.5
  zero10 : Constant  RequirementInfo={} %GIDa_596a5899_ba53_4c37_8272_7211e27ddf24
  zero9 : Constant  RequirementInfo={} %GIDa_b5c8c028_3d9d_45c0_afd9_41cf87627ef7  Value=0
  Out : Outport
  wires:
  Engage/1 -> Logical Operator5/1
  zero10/1 -> Logical Operator5/2
  zero9/1 -> Switch1/3
  In/1 -> Switch1/1
  Logical Operator5/1 -> Switch1/2
  Switch1/1 -> Out/1

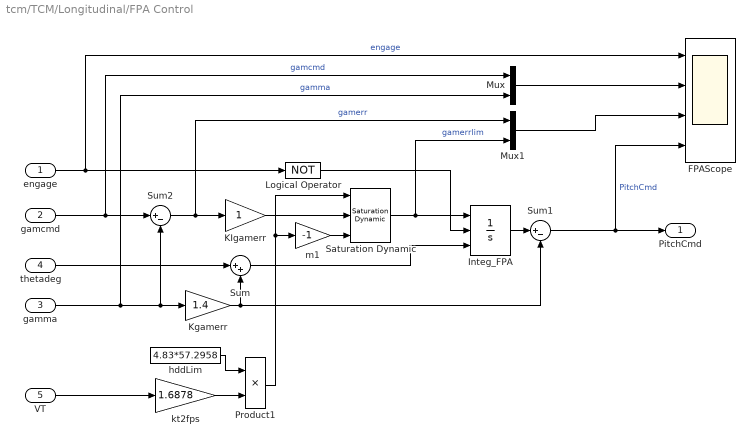
== system tcm/TCM/Longitudinal/FPA Control ==
  engage : Inport  RequirementInfo={} %GIDa_4330a6b4_8fd7_4be4_8132_0a5a51cb5321
  gamcmd : Inport  RequirementInfo={} %GIDa_72bd14a4_cf4e_4ddf_9979_bc189fd4e864  Port=2
  gamma : Inport  RequirementInfo={} %GIDa_07a290a4_e9be_4e9c_ae2b_d72f5ca4cb2b  Port=3
  thetadeg : Inport  RequirementInfo={} %GIDa_6ddd8d11_1197_4928_a2bc_231a82446ee7  Port=4
  VT : Inport  RequirementInfo={} %GIDa_a0a43ff9_fad6_4fc8_a8cd_c357b3dfb673  Port=5
  FPAScope : Scope  NumInputPorts=4
      settings: RequirementInfo={} %GIDa_08c55925_5efe_4d90_b09d_0072cafa98d7
  Integ_FPA : Integrator  RequirementInfo={} %GIDa_51acd94e_b58d_4d17_b07c_0b9ac17c0faa  ExternalReset=level  InitialConditionSource=external  IgnoreLimit=on
  KIgamerr : Gain  RequirementInfo={} %GIDa_08963e9e_c311_47c8_a63e_11cc7c9fb2d8
  Kgamerr : Gain  RequirementInfo={} %GIDa_3495b1a6_277d_4a6c_aa4f_649fc83b9092  Gain=1.4
  Logical Operator : Logic  RequirementInfo={} %GIDa_eba75fd0_479d_4894_b4e0_0ecea241815c  Operator=NOT  AllPortsSameDT=off  OutDataTypeStr=boolean
  Mux : Mux  RequirementInfo={} %GIDa_ae1e9d70_29ff_4004_97f5_396f2626ff0e  Inputs=2
  Mux1 : Mux  RequirementInfo={} %GIDa_b657458f_9c9c_48b1_af95_f550cfeae5f6  Inputs=2
  Product1 : Product  RequirementInfo={} %GIDa_bb863780_5e58_4e21_8791_e7a2c94dd786  RndMeth=Zero
  Saturation Dynamic : simulink/Discontinuities/Saturation Dynamic  OutMin=[]  OutMax=[]  OutDataTypeStr=Inherit: Same as second input  OutDataType=fixdt(1, 16)  OutScaling=2^-10  DoSatur=off
  Sum : Sum  RequirementInfo={} %GIDa_494c7255_4427_4dad_a3c1_4aee399936eb  Inputs=|++
  Sum1 : Sum  RequirementInfo={} %GIDa_93359946_60e9_438e_99e8_9beddee58b77  Inputs=|+-
  Sum2 : Sum  RequirementInfo={} %GIDa_c5e9feb7_f19d_4066_9b64_2fe045a465c2  Inputs=|+-
  hddLim : Constant  RequirementInfo={} %GIDa_1bf124ef_f3a0_4770_a704_52ef6436d4b5  Value=4.83*57.2958
  kt2fps : Gain  RequirementInfo={} %GIDa_c7ee5a6f_140d_48a3_b5c5_8ced7bef0603  Gain=1.6878
  m1 : Gain  RequirementInfo={} %GIDa_3e310fb8_58d1_4ad2_a1bc_b1914379a108  Gain=-1
  PitchCmd : Outport  RequirementInfo={} %GIDa_7e56bb7b_bd21_4466_8889_6a6d9858a2da
  wires:
  Sum1/1 -> PitchCmd/1, FPAScope/4  "PitchCmd"
  Kgamerr/1 -> Sum1/2, Sum/2
  Integ_FPA/1 -> Sum1/1
  gamma/1 -> Kgamerr/1, Sum2/2, Mux/2  "gamma"
  thetadeg/1 -> Sum/1
  Sum/1 -> Integ_FPA/3
  engage/1 -> Logical Operator/1, FPAScope/1  "engage"
  Logical Operator/1 -> Integ_FPA/2
  kt2fps/1 -> Product1/2
  hddLim/1 -> Product1/1
  Product1/1 -> Saturation Dynamic/1, m1/1
  VT/1 -> kt2fps/1
  Saturation Dynamic/1 -> Integ_FPA/1, Mux1/2  "gamerrlim"
  KIgamerr/1 -> Saturation Dynamic/2
  m1/1 -> Saturation Dynamic/3
  Sum2/1 -> KIgamerr/1, Mux1/1  "gamerr"
  gamcmd/1 -> Sum2/1, Mux/1  "gamcmd"
  Mux/1 -> FPAScope/2
  Mux1/1 -> FPAScope/3

== system tcm/TCM/Longitudinal/ManualOverride ==
  Man : Inport
  Auto : Inport  Port=2
  Switch1 : Switch  RequirementInfo={} %GIDa_891c72b6_c029_43c0_848a_219761f8f015  Criteria=u2 ~= 0  Threshold=0.5
  Out : Outport
  wires:
  Man/1 -> Switch1/3, Switch1/2
  Auto/1 -> Switch1/1
  Switch1/1 -> Out/1

== system tcm/TCM/Longitudinal/Pitch InnerLoop ==
  PitchCmd : Inport  RequirementInfo={} %GIDa_e681796d_a620_4c95_b4ed_ba3232dc70a2
  Pitch : Inport  RequirementInfo={} %GIDa_6f4baf24_a090_49e6_89b2_2ff3bd4fd377  Port=2
  qdeg : Inport  RequirementInfo={} %GIDa_13210493_e26c_4a14_89fc_8ad0299ca616  Port=3
  CAS : Inport  RequirementInfo={} %GIDa_e1a07f62_5dbf_46dc_bc2c_c2998ea01de8  Port=4
  Kcas : Lookup  RequirementInfo={} %GIDa_b4066843_ddd1_46cc_9bab_4de3e3ab273c  InputValues=[0 120 350 500]  Table=[1.0 1.0 0.3 0.3]
  Kpitch : Gain  RequirementInfo={} %GIDa_4a392bdb_3184_422c_b598_a156d3e8b02c  Gain=2
  Kwo : Gain  RequirementInfo={} %GIDa_6174b3c5_b132_42d6_a380_7a86f841c8e6  Gain=0.5
  Mux : Mux  RequirementInfo={} %GIDa_93279ee0_cc4a_4a25_b0b1_b731353743b0  Inputs=2
  PitchScope : Scope  NumInputPorts=6
      settings: RequirementInfo={} %GIDa_5646223d_16bd_44bf_9f51_c97977b5f9c0
  Product : Product  RequirementInfo={} %GIDa_ee2099f1_df06_4fc6_bf9b_0b7652de3a20  RndMeth=Zero
  Sum : Sum  RequirementInfo={} %GIDa_6e966264_2a04_4ed3_91bc_90c4039fd9a0  Inputs=|+-
  Sum1 : Sum  RequirementInfo={} %GIDa_5254d09e_07d7_42ec_bb70_93117997e359  Inputs=|-+
  Transfer Fcn : TransferFcn  RequirementInfo={} %GIDa_3bfe3d6e_47ed_45cd_9b22_d5337598ae49  Numerator=[16 0]  Denominator=[16 1]
  ElevCmd : Outport  RequirementInfo={} %GIDa_133d9978_a863_4cc3_b149_7ebb5beb5068
  wires:
  Sum/1 -> Kpitch/1, PitchScope/2  "Pitcherror"
  Pitch/1 -> Sum/2, Mux/2
  Kpitch/1 -> Sum1/1
  qdeg/1 -> Transfer Fcn/1
  Transfer Fcn/1 -> Kwo/1
  CAS/1 -> Kcas/1
  Sum1/1 -> Product/1, PitchScope/4  "dec"
  Kcas/1 -> Product/2, PitchScope/6  "Kcas"
  Product/1 -> ElevCmd/1, PitchScope/5  "elevcmd"
  Kwo/1 -> Sum1/2, PitchScope/3  "qdegwo"
  PitchCmd/1 -> Sum/1, Mux/1  "Pitchcmd"
  Mux/1 -> PitchScope/1

== system tcm/TCM/Yaw Damper/EngageORzero ==
  Engage : Inport
  In : Inport  Port=2
  Logical Operator5 : Logic  RequirementInfo={} %GIDa_039f8944_4af0_4d9a_b296_dc63f4fb9b24  AllPortsSameDT=off  OutDataTypeStr=boolean
  Switch1 : Switch  RequirementInfo={} %GIDa_5a57b0db_bac7_4f14_9c86_f79c8d73773a  Threshold=0.5
  zero10 : Constant  RequirementInfo={} %GIDa_459066bd_0987_4218_99ad_2fd246291f08
  zero9 : Constant  RequirementInfo={} %GIDa_11be025e_2612_434d_af1e_162a733bf0cc  Value=0
  Out : Outport
  wires:
  Engage/1 -> Logical Operator5/1
  zero10/1 -> Logical Operator5/2
  zero9/1 -> Switch1/3
  In/1 -> Switch1/1
  Logical Operator5/1 -> Switch1/2
  Switch1/1 -> Out/1

== system tcm/TCM/Yaw Damper/ManualOverride ==
  Man : Inport
  Auto : Inport  Port=2
  Switch1 : Switch  RequirementInfo={} %GIDa_c20200e4_a463_47a4_8bca_86ae3712d2e3  Criteria=u2 ~= 0  Threshold=0.5
  Out : Outport
  wires:
  Man/1 -> Switch1/3, Switch1/2
  Auto/1 -> Switch1/1
  Switch1/1 -> Out/1

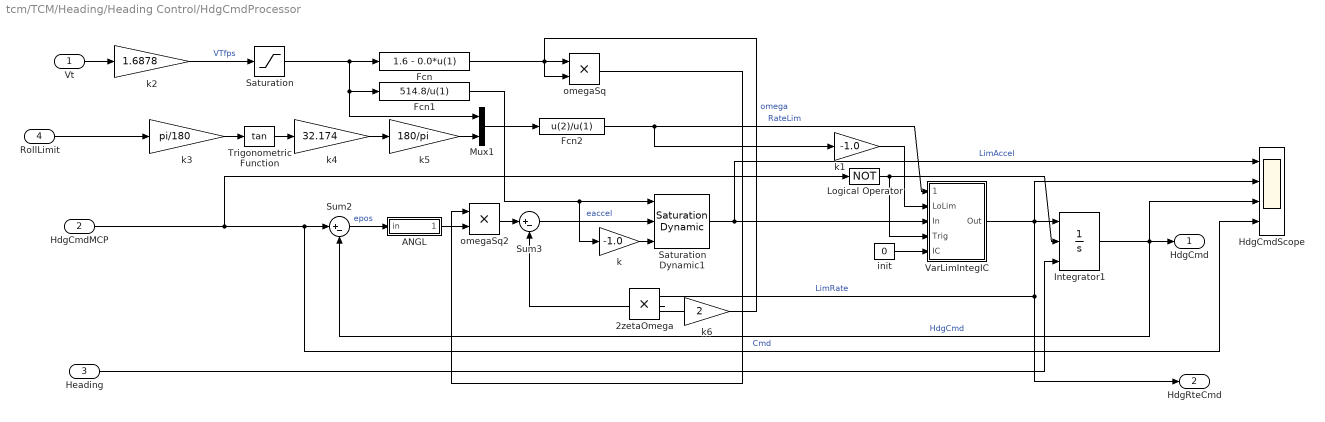
== system tcm/TCM/Heading/Heading Control/HdgCmdProcessor ==
  Vt : Inport  RequirementInfo={} %GIDa_aea371ad_7692_43c3_9333_237397a7088d
  HdgCmdMCP : Inport  RequirementInfo={} %GIDa_62146feb_aace_4fc2_8116_9e6cd7e3722f  Port=2
  Heading : Inport  RequirementInfo={} %GIDa_2367d888_2282_4a9b_9dc0_ce749bdb20fa  Port=3
  RollLimit : Inport  Port=4
  2zetaOmega : Product  RequirementInfo={} %GIDa_f321de1d_2313_4525_97dc_b8d5cf0673a7  RndMeth=Zero
  ANGL : Subsystem  RequirementInfo={} %GIDa_a65114d8_8cfa_43a6_b93e_efba84d5b466
  Fcn : Fcn  RequirementInfo={} %GIDa_4531d45e_6cbe_48a3_a177_15bd19e92740  Expr=1.6 - 0.0*u(1)
  Fcn1 : Fcn  RequirementInfo={} %GIDa_6e2df688_d84a_49b7_8178_2e4e2167c90a  Expr=514.8/u(1)
  Fcn2 : Fcn  RequirementInfo={} %GIDa_0806e265_28c4_47b9_a883_58ecb6812137  Expr=u(2)/u(1)
  HdgCmdScope : Scope  NumInputPorts=4
      settings: RequirementInfo={} %GIDa_44f9dfb2_1047_4c85_9993_6df91b14ae0d
  Integrator1 : Integrator  RequirementInfo={} %GIDa_fc49dfc1_f8ad_44f0_8a9e_cfbd72fa983d  ExternalReset=level  InitialConditionSource=external
  Logical Operator : Logic  RequirementInfo={} %GIDa_a3be1b8e_7e30_4ddb_8576_d6096a49c77e  Operator=NOT  AllPortsSameDT=off  OutDataTypeStr=boolean
  Mux1 : Mux  RequirementInfo={} %GIDa_fa4de243_ff79_4635_bf84_ab68fc6f4471  Inputs=2
  Saturation : Saturate  RequirementInfo={} %GIDa_34361c95_77fe_4878_a89a_f2e2245d083f  UpperLimit=1000  LowerLimit=0.0001
  Saturation Dynamic1 : simulink/Discontinuities/Saturation Dynamic  RequirementInfo={} %GIDa_3c1bb0e4_035b_467b_b908_73d0679fa8c4  OutMin=[]  OutMax=[]  OutDataTypeStr=Inherit: Same as second input  OutDataType=fixdt(1, 16)  OutScaling=2^-10  DoSatur=off
  Sum2 : Sum  RequirementInfo={} %GIDa_0134b7ed_8c9c_449a_ac58_c6bc449e5dc3  Inputs=|+-
  Sum3 : Sum  RequirementInfo={} %GIDa_133a47a4_a1d1_45cf_bb65_a8e707312c61  Inputs=|+-
  Trigonometric Function : Trigonometry  RequirementInfo={} %GIDa_9fedb248_844e_457e_a851_4a39016fb810  Operator=tan
  VarLimIntegIC : Subsystem  RequirementInfo={} %GIDa_5e236912_7c4b_441a_a6c7_d31391da156a
  init : Constant  RequirementInfo={} %GIDa_bb6a6882_f5a4_4f54_8f02_3d74a10327cc  Value=0
  k : Gain  RequirementInfo={} %GIDa_b3adcecb_db12_4f0e_a73c_fd191106ac98  Gain=-1.0
  k1 : Gain  RequirementInfo={} %GIDa_4080639b_e5dd_4b50_81e0_40e346cb6275  Gain=-1.0
  k2 : Gain  RequirementInfo={} %GIDa_3129ff2a_7a94_46f5_a52d_bf604afbaa9d  Gain=1.6878
  k3 : Gain  RequirementInfo={} %GIDa_bc42355c_264a_47e1_8506_c4c4e8e068fc  Gain=pi/180
  k4 : Gain  RequirementInfo={} %GIDa_0e3e2a32_c8b7_428f_ab0c_0faebbbf5e76  Gain=32.174
  k5 : Gain  RequirementInfo={} %GIDa_be5380e6_e279_4fba_b4a2_cea2808c46f4  Gain=180/pi
  k6 : Gain  RequirementInfo={} %GIDa_bccc5425_7281_49cf_93c6_a752e7732049  Gain=2
  omegaSq : Product  RequirementInfo={} %GIDa_e5c95743_58d1_4d7b_8e0f_0d5dca474f7a  RndMeth=Zero
  omegaSq2 : Product  RequirementInfo={} %GIDa_907b30dd_aede_4316_9a8a_044ea704cef8  RndMeth=Zero
  HdgCmd : Outport  RequirementInfo={} %GIDa_7c7f0b37_435d_4e7c_952c_62c879fcb657
  HdgRteCmd : Outport  RequirementInfo={} %GIDa_0b79bbaa_a2da_4cb9_814f_266c555013e7  Port=2
  wires:
  Integrator1/1 -> Sum2/2, HdgCmd/1, HdgCmdScope/3  "HdgCmd"
  Vt/1 -> k2/1
  k2/1 -> Saturation/1  "VTfps"
  Fcn/1 -> omegaSq/2, omegaSq/1, k6/1  "omega"
  k/1 -> Saturation Dynamic1/3
  Mux1/1 -> Fcn2/1
  RollLimit/1 -> k3/1
  Sum3/1 -> Saturation Dynamic1/2  "eaccel"
  Saturation Dynamic1/1 -> VarLimIntegIC/3(In), HdgCmdScope/1  "LimAccel"
  k3/1 -> Trigonometric Function/1
  Trigonometric Function/1 -> k4/1
  k4/1 -> k5/1
  k5/1 -> Mux1/2
  Fcn2/1 -> VarLimIntegIC/1(UpLim), k1/1  "RateLim"
  k1/1 -> VarLimIntegIC/2(LoLim)
  VarLimIntegIC/1(Out) -> Integrator1/1, HdgCmdScope/2, 2zetaOmega/1, HdgRteCmd/1  "LimRate"
  k6/1 -> 2zetaOmega/2
  2zetaOmega/1 -> Sum3/2
  Fcn1/1 -> k/1, Saturation Dynamic1/1
  init/1 -> VarLimIntegIC/5(IC)
  omegaSq/1 -> omegaSq2/1
  omegaSq2/1 -> Sum3/1
  Sum2/1 -> ANGL/1(in)  "epos"
  HdgCmdMCP/1 -> Logical Operator/1, Sum2/1, HdgCmdScope/4  "Cmd"
  ANGL/1(+ -180) -> omegaSq2/2
  Logical Operator/1 -> VarLimIntegIC/4(Trig), Integrator1/2
  Saturation/1 -> Fcn/1, Mux1/1, Fcn1/1
  Heading/1 -> Integrator1/3

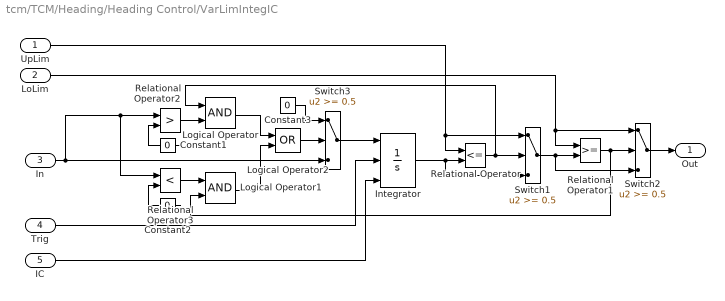
== system tcm/TCM/Heading/Heading Control/VarLimIntegIC ==
  UpLim : Inport  RequirementInfo={} %GIDa_a52f7b7f_3cd2_4b84_aa46_8f49d190de5c
  LoLim : Inport  RequirementInfo={} %GIDa_14f49477_0466_41ac_a405_ff8b353df89c  Port=2
  In : Inport  RequirementInfo={} %GIDa_3e285f49_2930_4df4_81dd_a9b406bbe3bd  Port=3
  Trig : Inport  RequirementInfo={} %GIDa_a10733bc_08b5_4d2b_a4b2_d21b5a57b6cc  Port=4
  IC : Inport  RequirementInfo={} %GIDa_1f0c5f5f_64dd_4362_ac43_aa1a0320c078  Port=5
  Constant1 : Constant  RequirementInfo={} %GIDa_06ecceb0_a33e_4777_98b5_cbb205f23b1a  Value=0
  Constant2 : Constant  RequirementInfo={} %GIDa_450747a0_c4d7_4d05_b9cd_637cc0a6e70e  Value=0
  Constant3 : Constant  RequirementInfo={} %GIDa_2162f9e8_6490_497e_a11b_22bba3b34cf8  Value=0
  Integrator : Integrator  RequirementInfo={} %GIDa_1e518e6b_aff4_4186_bd69_b47d2c7ff727  ExternalReset=level  InitialConditionSource=external
  Logical Operator : Logic  RequirementInfo={} %GIDa_08f35c7f_9ec6_4cc6_9a1f_42b21408c66a  AllPortsSameDT=off
  Logical Operator1 : Logic  RequirementInfo={} %GIDa_78d08ac2_a159_4fb8_990a_70ef898240f1  AllPortsSameDT=off
  Logical Operator2 : Logic  RequirementInfo={} %GIDa_16203443_42bb_4de7_9e01_30a8f399b69b  Operator=OR  AllPortsSameDT=off
  Relational Operator : RelationalOperator  RequirementInfo={} %GIDa_fd2b09f2_7292_41cd_b490_47957a93b770  Operator=<=
  Relational Operator1 : RelationalOperator  RequirementInfo={} %GIDa_bc21e44d_a4ad_4459_a4e5_c40c404b3dbb
  Relational Operator2 : RelationalOperator  RequirementInfo={} %GIDa_257b199b_80e3_40b3_851a_c63ec13dd9de  Operator=>
  Relational Operator3 : RelationalOperator  RequirementInfo={} %GIDa_34126d1c_0a68_4b2a_a8f9_adf647778def  Operator=<
  Switch1 : Switch  RequirementInfo={} %GIDa_093ada51_26d0_4dd4_951b_93ea95402387  Threshold=0.5  SaturateOnIntegerOverflow=on  InputSameDT=on
  Switch2 : Switch  RequirementInfo={} %GIDa_ce0381f3_056e_496f_90b9_8ff8975dbd4b  Threshold=0.5  SaturateOnIntegerOverflow=on  InputSameDT=on
  Switch3 : Switch  RequirementInfo={} %GIDa_23ed59f4_3b4c_47cd_8936_54e05a064030  Threshold=0.5  SaturateOnIntegerOverflow=on  InputSameDT=on
  Out : Outport  RequirementInfo={} %GIDa_a2a80f39_47d8_4649_81f4_5246420c0c65
  wires:
  Relational Operator1/1 -> Logical Operator1/2, Switch2/2
  Switch1/1 -> Switch2/3, Relational Operator1/2
  LoLim/1 -> Relational Operator1/1, Switch2/1
  IC/1 -> Integrator/3
  Trig/1 -> Integrator/2
  Constant2/1 -> Relational Operator3/2
  Relational Operator3/1 -> Logical Operator1/1
  Logical Operator1/1 -> Logical Operator2/2
  Logical Operator/1 -> Logical Operator2/1
  Logical Operator2/1 -> Switch3/2
  Relational Operator2/1 -> Logical Operator/2
  Constant1/1 -> Relational Operator2/2
  In/1 -> Switch3/3, Relational Operator3/1, Relational Operator2/1
  Constant3/1 -> Switch3/1
  Switch3/1 -> Integrator/1
  Relational Operator/1 -> Logical Operator/1, Switch1/2
  Switch2/1 -> Out/1
  UpLim/1 -> Switch1/1, Relational Operator/1
  Integrator/1 -> Relational Operator/2, Switch1/3

== system tcm/TCM/Longitudinal/Altitude Control/Variable  Rate Limit ==
  ratelim : Inport  RequirementInfo={} %GIDa_1ef85aab_f902_404e_a68b_00e57673dd3f
  input : Inport  RequirementInfo={} %GIDa_7ac59940_1fcc_4039_a5aa_a007950c590e  Port=2
  ICtrig : Inport  RequirementInfo={} %GIDa_9850dee7_08ca_49d5_88fb_399ee4ba203e  Port=3
  IC : Inport  RequirementInfo={} %GIDa_d80fe626_91fd_4f82_ad17_86aca6b3aee5  Port=4
  Gain : Gain  RequirementInfo={} %GIDa_55467e41_3bd6_44bf_9a44_6f78661bf8f0  Gain=20  SaturateOnIntegerOverflow=on  OutDataTypeStr=Inherit: Same as input  ParamDataTypeStr=Inherit: Same as input
  Gain1 : Gain  RequirementInfo={} %GIDa_0b7dd2e9_dfcf_42d3_8fb1_8c254e005ceb  Gain=-1  SaturateOnIntegerOverflow=on  OutDataTypeStr=Inherit: Same as input  ParamDataTypeStr=Inherit: Same as input
  Integrator : Integrator  RequirementInfo={} %GIDa_e056ed2c_99cd_43ff_ba72_481853046efe  ExternalReset=level  InitialConditionSource=external  IgnoreLimit=on
  Sum2 : Sum  RequirementInfo={} %GIDa_de9ff84b_54f5_48bc_9ef3_874415208380  Inputs=|+-  SaturateOnIntegerOverflow=on
  Variable Limit Saturation : Subsystem  RequirementInfo={} %GIDa_42540829_63e9_4d83_adf5_d7c684208c2d
  output : Outport  RequirementInfo={} %GIDa_74eb2916_410f_4b2d_afdf_0d476e7e03b7
  wires:
  Sum2/1 -> Gain/1
  Gain/1 -> Variable Limit Saturation/2(SigIn)
  ratelim/1 -> Gain1/1, Variable Limit Saturation/1(up_lim)
  Gain1/1 -> Variable Limit Saturation/3(Lo_lim)
  Variable Limit Saturation/1(Out1) -> Integrator/1
  Integrator/1 -> Sum2/2, output/1
  input/1 -> Sum2/1
  ICtrig/1 -> Integrator/2
  IC/1 -> Integrator/3

== system tcm/TCM/Longitudinal/Altitude Control/Variable Limit Saturation ==
  up_lim : Inport  RequirementInfo={} %GIDa_a8c5a358_1294_4ae6_a63f_3940fe218386
  SigIn : Inport  RequirementInfo={} %GIDa_062a0af8_40f0_4204_856b_8e0aded8de05  Port=2
  Lo_lim : Inport  RequirementInfo={} %GIDa_6793747b_c094_4bd9_a5cb_839f8eb54e21  Port=3
  Enforce low lim : MinMax  RequirementInfo={} %GIDa_e93f4b97_2f8b_4f52_84c9_3cb68ddf7e16  Function=max  Inputs=2
  Enforce up lim : MinMax  RequirementInfo={} %GIDa_c018e6ad_c664_4361_a96c_d990e2efb7d8  Inputs=2
  Out1 : Outport  RequirementInfo={} %GIDa_0d7a9d35_dde5_41a4_a708_f2de214bfa54
  wires:
  Lo_lim/1 -> Enforce low lim/1
  SigIn/1 -> Enforce low lim/2
  Enforce low lim/1 -> Enforce up lim/1
  up_lim/1 -> Enforce up lim/2
  Enforce up lim/1 -> Out1/1

== system tcm/TCM/Heading/Heading Control/HdgCmdProcessor/ANGL ==
  in : Inport  RequirementInfo={} %GIDa_91f853c7_c908_401d_adfc_518d7751528f
  Constant1 : Constant  RequirementInfo={} %GIDa_7c5c3c02_b72b_4cab_88d9_ce8964dea6e5  Value=180
  Fcn1 : Fcn  RequirementInfo={} %GIDa_213b457a_3bda_40ee_98ea_3904c5a57eac  Expr=360*sgn(u(1))
  Fcn2 : Fcn  RequirementInfo={} %GIDa_e30acbdf_c224_4031_bd02_e86b06b14b6c  Expr=abs(u(1))
  Relational Operator : RelationalOperator  RequirementInfo={} %GIDa_7fca63f4_30c3_4611_a13c_f242258541ac  Operator=>
  Sum6 : Sum  RequirementInfo={} %GIDa_8f691f86_6b2c_4343_a08d_01121fff99a8  Inputs=|-+  SaturateOnIntegerOverflow=on
  Switch1 : Switch  RequirementInfo={} %GIDa_9f6a3e17_ac1f_4a7c_b770_43e31d539b0d  Threshold=0.1  SaturateOnIntegerOverflow=on
  + -180 : Outport  RequirementInfo={} %GIDa_da671ccf_1469_4f90_9911_e50416dafc2f
  wires:
  Fcn2/1 -> Relational Operator/1
  in/1 -> Switch1/3, Sum6/2, Fcn1/1, Fcn2/1
  Switch1/1 -> + -180/1
  Fcn1/1 -> Sum6/1
  Sum6/1 -> Switch1/1
  Relational Operator/1 -> Switch1/2
  Constant1/1 -> Relational Operator/2

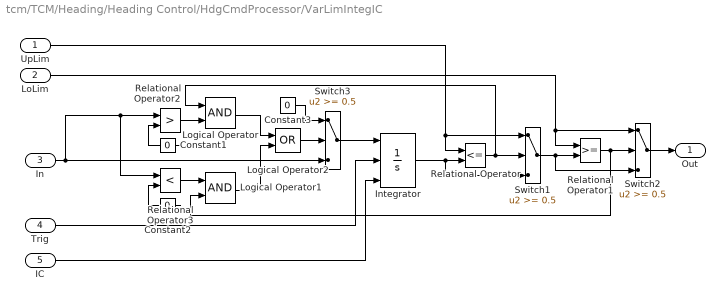
== system tcm/TCM/Heading/Heading Control/HdgCmdProcessor/VarLimIntegIC ==
  UpLim : Inport  RequirementInfo={} %GIDa_b6974814_32b4_446c_a7b5_2b64616822d2
  LoLim : Inport  RequirementInfo={} %GIDa_b4069f0f_04d2_435d_9d74_47f31e226abc  Port=2
  In : Inport  RequirementInfo={} %GIDa_ffe63698_9663_4b08_a6c4_0cfcc14ab018  Port=3
  Trig : Inport  RequirementInfo={} %GIDa_6297cb9d_5b31_4d8e_a321_41fbf142c5b4  Port=4
  IC : Inport  RequirementInfo={} %GIDa_59f2d505_3cc2_4942_9dd8_a5a4ff923eba  Port=5
  Constant1 : Constant  RequirementInfo={} %GIDa_5f63bf18_9b52_4c75_b33f_d083ba316d1e  Value=0
  Constant2 : Constant  RequirementInfo={} %GIDa_3ef1a0c3_325a_4a1e_87f1_8a7ceb7f2ed7  Value=0
  Constant3 : Constant  RequirementInfo={} %GIDa_3c010cc6_e66d_42da_9a5a_231ebe5e9c3f  Value=0
  Integrator : Integrator  RequirementInfo={} %GIDa_f7b1bc6b_014b_45d2_839c_eec18249e41d  ExternalReset=level  InitialConditionSource=external
  Logical Operator : Logic  RequirementInfo={} %GIDa_a60b4d2f_6552_4cb5_b522_727de66498b0  AllPortsSameDT=off
  Logical Operator1 : Logic  RequirementInfo={} %GIDa_8f81d6cf_a2aa_4e00_869d_ceffbd7871c1  AllPortsSameDT=off
  Logical Operator2 : Logic  RequirementInfo={} %GIDa_6338745d_e0be_46bf_a46f_644f808dad4e  Operator=OR  AllPortsSameDT=off
  Relational Operator : RelationalOperator  RequirementInfo={} %GIDa_8e878cd0_b3b2_4162_9fe2_c686049f0806  Operator=<=
  Relational Operator1 : RelationalOperator  RequirementInfo={} %GIDa_b45a0ded_1a8c_4a6d_a67f_e5d263373459
  Relational Operator2 : RelationalOperator  RequirementInfo={} %GIDa_a0755ed8_a69f_4262_8ce5_c41fc56502ff  Operator=>
  Relational Operator3 : RelationalOperator  RequirementInfo={} %GIDa_8264758e_f6c1_4924_85b8_a6eda5126d21  Operator=<
  Switch1 : Switch  RequirementInfo={} %GIDa_4c3fce01_41f9_40b1_a6a3_6d04c9eccd5a  Threshold=0.5  SaturateOnIntegerOverflow=on  InputSameDT=on
  Switch2 : Switch  RequirementInfo={} %GIDa_b2e7bf7c_7029_45e6_9cda_915a12f41445  Threshold=0.5  SaturateOnIntegerOverflow=on  InputSameDT=on
  Switch3 : Switch  RequirementInfo={} %GIDa_bec6d583_cd7d_4a0e_9481_7e8d505e2b66  Threshold=0.5  SaturateOnIntegerOverflow=on  InputSameDT=on
  Out : Outport  RequirementInfo={} %GIDa_6b54eae4_0c2d_43e8_87f0_b15564168c0d
  wires:
  Relational Operator1/1 -> Logical Operator1/2, Switch2/2
  Switch1/1 -> Switch2/3, Relational Operator1/2
  LoLim/1 -> Relational Operator1/1, Switch2/1
  IC/1 -> Integrator/3
  Trig/1 -> Integrator/2
  Constant2/1 -> Relational Operator3/2
  Relational Operator3/1 -> Logical Operator1/1
  Logical Operator1/1 -> Logical Operator2/2
  Logical Operator/1 -> Logical Operator2/1
  Logical Operator2/1 -> Switch3/2
  Relational Operator2/1 -> Logical Operator/2
  Constant1/1 -> Relational Operator2/2
  In/1 -> Switch3/3, Relational Operator3/1, Relational Operator2/1
  Constant3/1 -> Switch3/1
  Switch3/1 -> Integrator/1
  Relational Operator/1 -> Logical Operator/1, Switch1/2
  Switch2/1 -> Out/1
  UpLim/1 -> Switch1/1, Relational Operator/1
  Integrator/1 -> Relational Operator/2, Switch1/3

== system tcm/TCM/Longitudinal/Altitude Control/Variable  Rate Limit/Variable Limit Saturation ==
  up_lim : Inport  RequirementInfo={} %GIDa_c3426702_ae57_4a6b_8e5b_d8e7ea7997b8
  SigIn : Inport  RequirementInfo={} %GIDa_57ffe4bd_514b_4f1d_925b_ea07d6710330  Port=2
  Lo_lim : Inport  RequirementInfo={} %GIDa_934c3ebb_c2a8_4cb2_b1d4_7a7b38287908  Port=3
  Enforce low lim : MinMax  RequirementInfo={} %GIDa_f320f771_b833_4e25_ab12_e91693dd9b04  Function=max  Inputs=2
  Enforce up lim : MinMax  RequirementInfo={} %GIDa_1cfdde9a_faa1_4e7e_9516_cacb3f0cb773  Inputs=2
  Out1 : Outport  RequirementInfo={} %GIDa_6b324e36_3b21_43eb_ae92_bdd39356922a
  wires:
  Enforce up lim/1 -> Out1/1
  up_lim/1 -> Enforce up lim/2
  Enforce low lim/1 -> Enforce up lim/1
  SigIn/1 -> Enforce low lim/2
  Lo_lim/1 -> Enforce low lim/1
